simulink model "charging_pile"  (Simulink 7.6)
settings: Solver=ode23tb  StartTime=0.0  StopTime=0.2  RelTol=1e-3
libraries: powerlib x22, powerlib_extras x2, simulink x1
settings Model: Creator=Administrator  LastModifiedBy=Administrator
settings SimEventsCC: propDiagAttribOutput=1  propDiagFcnCallOutput=1  propDiagStatOutput=0

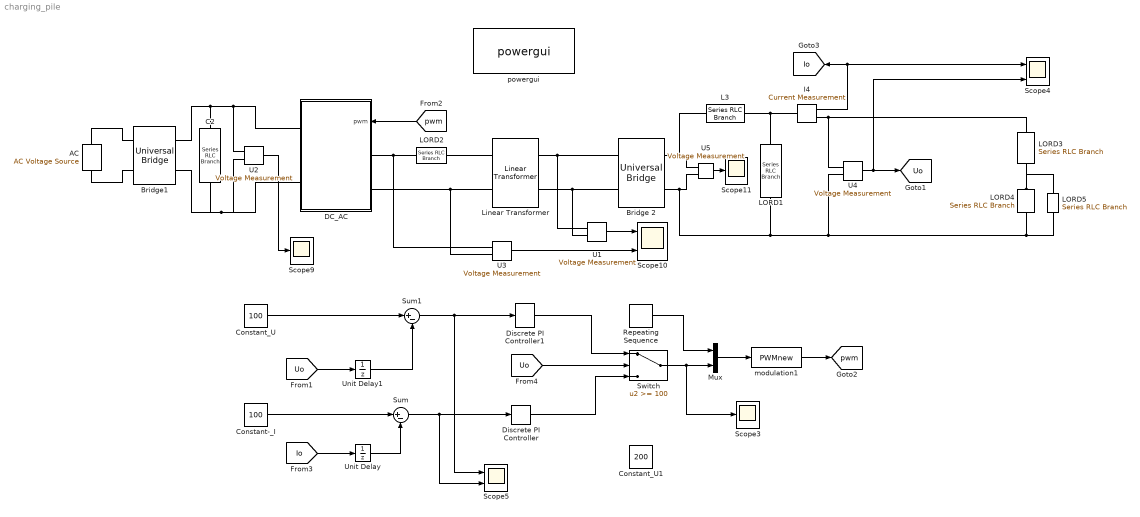
== system charging_pile ==
  " Bridge 2" : powerlib/Power Electronics/Universal Bridge  DialogController=POWERSYS.PowerSysDialog  SystemSampleTime=-1  Arms=2  SnubberResistance=5  SnubberCapacitance=1e-5  Device=Diodes  Ron=1e-3  Lon=0  ForwardVoltages="[  0  0  ]"  ForwardVoltage=0  GTOparameters=[ 10e-6 , 20e-6 ]  IGBTparameters=[ 1e-6 , 2e-6 ]  Measurements=None  Measurements_2=None  converterType=Rectifier
  " Bridge1" : powerlib/Power Electronics/Universal Bridge  DialogController=POWERSYS.PowerSysDialog  SystemSampleTime=-1  Arms=2  SnubberResistance=5  SnubberCapacitance=1e-5  Device=Diodes  Ron=1e-3  Lon=0  ForwardVoltages="[  0  0  ]"  ForwardVoltage=0  GTOparameters=[ 10e-6 , 20e-6 ]  IGBTparameters=[ 1e-6 , 2e-6 ]  Measurements=None  Measurements_2=None  converterType=Rectifier
  "AC " : powerlib/Electrical Sources/AC Voltage Source  DialogController=POWERSYS.PowerSysDialog  SystemSampleTime=-1  Amplitude=311  Phase=0  Frequency=50  SampleTime=0  Measurements=None
  C2 : powerlib/Elements/Series RLC Branch  DialogController=POWERSYS.PowerSysDialog  PhysicalDomain=powersysdomain  SubClassName=unknown  LeftPortType=p1  RightPortType=p1  LConnTagsString=__new0  RConnTagsString=__new0  BranchType=C  Resistance=0.001  Inductance=1e-3  SetiL0=off  InitialCurrent=0  Capacitance=20000e-6  Setx0=on  InitialVoltage=0  Measurements=None
  Constant-_I : Constant  Value=100
  Constant_U : Constant  Value=100
  Constant_U1 : Constant  Value=200
  DC_AC : Subsystem
  Discrete PI Controller : powerlib_extras/Discrete  Control Blocks/Discrete PI Controller  DialogController=POWERSYS.PowerSysDialog  SystemSampleTime=-1  Kp=1000  Ki=100  Par_Limits=[2700 100]  Init=100  Ts=2e-6
  Discrete PI Controller1 : powerlib_extras/Discrete  Control Blocks/Discrete PI Controller  DialogController=POWERSYS.PowerSysDialog  SystemSampleTime=-1  Kp=1000  Ki=100  Par_Limits=[2700 100]  Init=100  Ts=2e-6
  I4 : powerlib/Measurements/Current Measurement  DialogController=POWERSYS.PowerSysDialog  SystemSampleTime=-1  PhasorSimulation=off  OutputType=Complex  PSBequivalent=0
  L3 : powerlib/Elements/Series RLC Branch  DialogController=POWERSYS.PowerSysDialog  PhysicalDomain=powersysdomain  SubClassName=unknown  LeftPortType=p1  RightPortType=p1  LConnTagsString=__new0  RConnTagsString=__new0  BranchType=L  Resistance=1  Inductance=1e-3  SetiL0=off  InitialCurrent=0  Capacitance=4000e-6  Setx0=off  InitialVoltage=0  Measurements=None
  LORD1 : powerlib/Elements/Series RLC Branch  DialogController=POWERSYS.PowerSysDialog  PhysicalDomain=powersysdomain  SubClassName=unknown  LeftPortType=p1  RightPortType=p1  LConnTagsString=__new0  RConnTagsString=__new0  BranchType=C  Resistance=0.01  Inductance=1e-3  SetiL0=off  InitialCurrent=0  Capacitance=25e-6  Setx0=off  InitialVoltage=0  Measurements=None
  LORD2 : powerlib/Elements/Series RLC Branch  DialogController=POWERSYS.PowerSysDialog  PhysicalDomain=powersysdomain  SubClassName=unknown  LeftPortType=p1  RightPortType=p1  LConnTagsString=__new0  RConnTagsString=__new0  BranchType=C  Resistance=0.01  Inductance=1e-3  SetiL0=off  InitialCurrent=0  Capacitance=60e-6  Setx0=off  InitialVoltage=0  Measurements=None
  LORD3 : powerlib/Elements/Series RLC Branch  DialogController=POWERSYS.PowerSysDialog  PhysicalDomain=powersysdomain  SubClassName=unknown  LeftPortType=p1  RightPortType=p1  LConnTagsString=__new0  RConnTagsString=__new0  BranchType=R  Resistance=0.1  Inductance=1e-3  SetiL0=off  InitialCurrent=0  Capacitance=50000e-6  Setx0=off  InitialVoltage=0  Measurements=None
  LORD4 : powerlib/Elements/Series RLC Branch  DialogController=POWERSYS.PowerSysDialog  PhysicalDomain=powersysdomain  SubClassName=unknown  LeftPortType=p1  RightPortType=p1  LConnTagsString=__new0  RConnTagsString=__new0  BranchType=C  Resistance=0.1  Inductance=1e-3  SetiL0=off  InitialCurrent=0  Capacitance=0.1  Setx0=off  InitialVoltage=50  Measurements=None
  LORD5 : powerlib/Elements/Series RLC Branch  DialogController=POWERSYS.PowerSysDialog  PhysicalDomain=powersysdomain  SubClassName=unknown  LeftPortType=p1  RightPortType=p1  LConnTagsString=__new0  RConnTagsString=__new0  BranchType=R  Resistance=25  Inductance=1e-3  SetiL0=off  InitialCurrent=0  Capacitance=50000e-6  Setx0=off  InitialVoltage=0  Measurements=None
  Linear Transformer : powerlib/Elements/Linear Transformer  DialogController=POWERSYS.PowerSysDialog  PhysicalDomain=powersysdomain  SubClassName=unknown  LeftPortType=p1  RightPortType=p1  LConnTagsString=a|b  RConnTagsString=A|B  UNITS=SI  NominalPower=[ 15e3 20000 ]  winding1=[311 0.0064481 2.0525e-006]  winding2=[173 0.0019953 6.3511e-007]  ThreeWindings=off  winding3=[3.15e+005 6615 2.1056]  RmLm=[1612 0.012828]  Measurements=None  DataType=on
  Mux : Mux  Inputs=2
  Repeating Sequence : simulink/Sources/Repeating Sequence  SystemSampleTime=-1  rep_seq_t=[0 1/1e4]  rep_seq_y=[0 6000]
  Scope10 : Scope  NumInputPorts=2
      settings: TimeRange=0.2  YMin=-400~-5  YMax=400~5  SaveName=ScopeData9  MaxDataPoints=10000000
  Scope11 : Scope
      settings: TimeRange=0.04000000000000001  YMin=-700  YMax=700  SaveName=ScopeData10  MaxDataPoints=10000000
  Scope3 : Scope
      settings: TimeRange=0.04000000000000001  YMin=-700  YMax=700  SaveName=ScopeData2  MaxDataPoints=10000000
  Scope4 : Scope  NumInputPorts=2
      settings: TimeRange=0.04000000000000001  YMin=0~86  YMax=100~101  SaveName=ScopeData3  MaxDataPoints=10000000
  Scope5 : Scope  NumInputPorts=2
      settings: TimeRange=0.04000000000000001  YMin=-2.5~30  YMax=30~100  SaveName=ScopeData4  MaxDataPoints=10000000
  Scope9 : Scope
      settings: TimeRange=0.04000000000000001  YMin=267.5  YMax=312.5  SaveName=ScopeData8  MaxDataPoints=10000000
  Sum : Sum  Inputs=|+-
  Sum1 : Sum  Inputs=|+-
  Switch : Switch  Threshold=100
  U{1..5} (5 alike) : powerlib/Measurements/Voltage Measurement  DialogController=POWERSYS.PowerSysDialog  SystemSampleTime=-1  PhasorSimulation=off  OutputType=Complex  PSBequivalent=0
  Unit Delay : UnitDelay  SampleTime=-1
  Unit Delay1 : UnitDelay  SampleTime=-1
  modulation1 : S-Function  FunctionName=PWMnew  EnableBusSupport=off
  powergui : powerlib/powergui  Priority=1  SystemSampleTime=-1  SimulationMode=Discrete  SampleTime=2e-6  frequency=60  SPID=off  DisableSnubberDevices=off  DisableRonSwitches=off  DisableVfSwitches=off  SwTol=0  Interpol=off  frequencyindice=0  echomessages=off  HookPort=off  DisplayEquations=off  FunctionMessages=off  EnableUseOfTLC=off  x0status=blocks  RestoreLinks=warning  ResistiveCurrentMeasurement=off  Frange=[0:2:500]  Ylog=off  Xlog=on  ShowGrid=off  save=off  variable=ZData  structure=ScopeData2  ZoomFFT=off  StartTime=0.04  cycles=2  DisplayStyle=1  fundamental=50  FreqAxis=on  MaxFrequency=1000  frequencyindicesteady=1  RmsSteady=1  display=off  Ts=0  methode=off
  tag scope: Io=global, Uo=global, pwm=global
  wires:
  Constant-_I/1 -> Sum/1
  [Io] -> Unit Delay/1
  Constant_U/1 -> Sum1/1
  [Uo] -> Unit Delay1/1
  Sum/1 -> Discrete PI Controller/1, Scope5/2
  Sum1/1 -> Discrete PI Controller1/1, Scope5/1
  I4/1 -> [Io], Scope4/1
  U4/1 -> [Uo], Scope4/2
  Unit Delay/1 -> Sum/2
  Unit Delay1/1 -> Sum1/2
  [pwm] -> DC_AC/1(pwm)
  [Uo] -> Switch/2
  Discrete PI Controller1/1 -> Switch/1
  Discrete PI Controller/1 -> Switch/3
  U2/1 -> Scope9/1
  U5/1 -> Scope11/1
  Repeating Sequence/1 -> Mux/1
  Mux/1 -> modulation1/1
  modulation1/1 -> [pwm]
  U3/1 -> Scope10/2
  U1/1 -> Scope10/1
  Switch/1 -> Mux/2, Scope3/1
  connections:
  " Bridge 2"/LConn2 -- Linear Transformer/RConn2 -- U1/LConn2
  L3/LConn1 -- I4/LConn1 -- LORD1/LConn1
  " Bridge 2"/LConn1 -- Linear Transformer/RConn1 -- U1/LConn1
  "AC "/RConn1 -- " Bridge1"/LConn1
  "AC "/LConn1 -- " Bridge1"/LConn2
  U5/LConn1 -- L3/RConn1 -- " Bridge 2"/RConn1
  I4/RConn1 -- U4/LConn1 -- LORD3/LConn1
  DC_AC/RConn1 -- C2/LConn1 -- " Bridge1"/RConn1 -- U2/LConn1
  C2/RConn1 -- " Bridge1"/RConn2 -- DC_AC/RConn2 -- U2/LConn2
  " Bridge 2"/RConn2 -- U5/LConn2 -- LORD1/RConn1 -- LORD5/RConn1 -- LORD4/RConn1 -- U4/LConn2
  LORD2/LConn1 -- DC_AC/LConn1 -- U3/LConn1
  DC_AC/LConn2 -- Linear Transformer/LConn2 -- U3/LConn2
  LORD3/RConn1 -- LORD4/LConn1 -- LORD5/LConn1
  Linear Transformer/LConn1 -- LORD2/RConn1

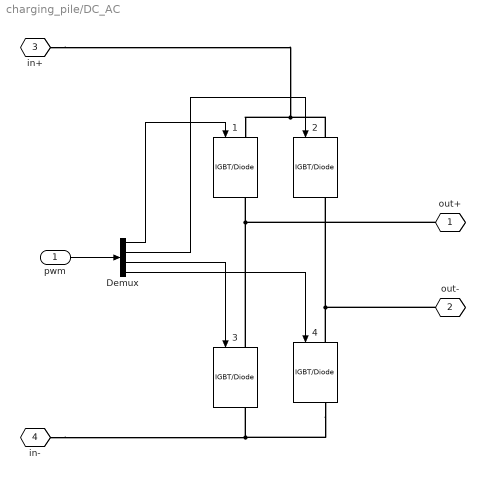
== system charging_pile/DC_AC ==
  pwm : Inport
  1 : powerlib/Power Electronics/IGBT//Diode  DialogController=POWERSYS.PowerSysDialog  SystemSampleTime=-1  Ron=1e-3  Rs=1e4  Cs=0.1e-6  Measurements=on
  2 : powerlib/Power Electronics/IGBT//Diode  DialogController=POWERSYS.PowerSysDialog  SystemSampleTime=-1  Ron=1e-3  Rs=1e4  Cs=100e-9  Measurements=on
  3 : powerlib/Power Electronics/IGBT//Diode  DialogController=POWERSYS.PowerSysDialog  SystemSampleTime=-1  Ron=1e-3  Rs=1e4  Cs=100e-9  Measurements=on
  4 : powerlib/Power Electronics/IGBT//Diode  DialogController=POWERSYS.PowerSysDialog  SystemSampleTime=-1  Ron=1e-3  Rs=1e4  Cs=100e-9  Measurements=on
  Demux : Demux
  out+ : PMIOPort  Tag=PMCPort  Port=1  Side=Left
  out- : PMIOPort  Tag=PMCPort  Port=2  Side=Left
  in+ : PMIOPort  Tag=PMCPort  Port=3  Side=Right
  in- : PMIOPort  Tag=PMCPort  Port=4  Side=Right
  wires:
  Demux/1 -> 1/1
  Demux/2 -> 2/1
  Demux/3 -> 3/1
  Demux/4 -> 4/1
  pwm/1 -> Demux/1
  connections:
  4/RConn1 -- 3/RConn1 -- in-/RConn1
  4/LConn1 -- 2/RConn1 -- out-/RConn1
  3/LConn1 -- 1/RConn1 -- out+/RConn1
  2/LConn1 -- 1/LConn1 -- in+/RConn1
